simulink model "Ex1"  (R2023a)
settings: Solver=VariableStepAuto  StartTime=0.0  StopTime=10.0  RelTol=1e-3
settings Model: Creator=Aman  LastModifiedBy=Aman

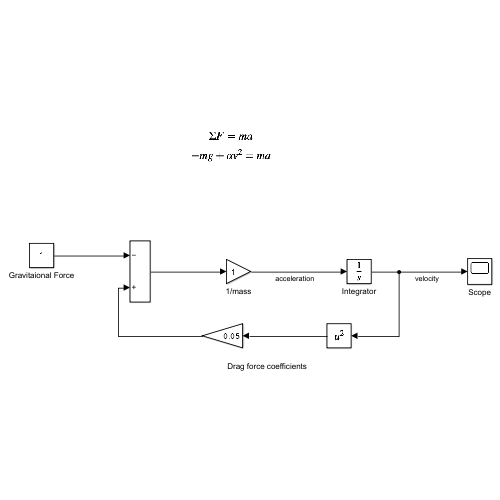
[thumbnail: Simulink's stored preview of the top-level diagram]
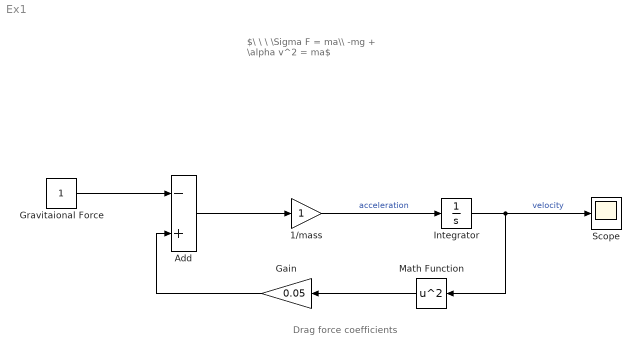
== system Ex1 ==
  note: Drag force coefficients
  note: $\ \ \ \Sigma F = ma\\ -mg + \alpha v^2 = ma$
  1/mass : Gain
  Add : Sum  Inputs=-+
  Gain : Gain  Gain=0.05
  Gravitaional Force : Constant
  Integrator : Integrator
  Math Function : Math  Operator=square
  Scope : Scope
  wires:
  Gravitaional Force/1 -> Add/1
  Add/1 -> 1/mass/1
  1/mass/1 -> Integrator/1  "acceleration"
  Integrator/1 -> Math Function/1, Scope/1  "velocity"
  Math Function/1 -> Gain/1
  Gain/1 -> Add/2
